simulink model "BMSOut"  (R2024b)
settings: configuration reference "VehicleFixed100ms" (kept outside this file)
undefined symbols (not defined in the file): PlntBattNumCellSer
settings Model: DataDictionary=VirtualVehicleTemplate.sldd  ModifiedByFormat=The MathWorks, Inc.  ExtModeTrigDuration=5  Creator=The MathWorks, Inc.  LastModifiedBy=The MathWorks, Inc.
settings ConfigSetRef: SourceName=VehicleFixed100ms

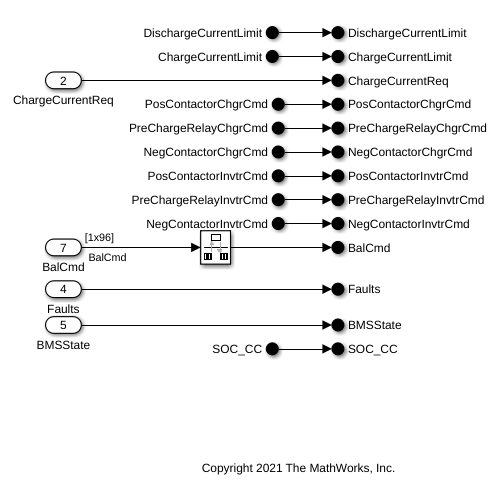
[thumbnail: Simulink's stored preview of the top-level diagram]
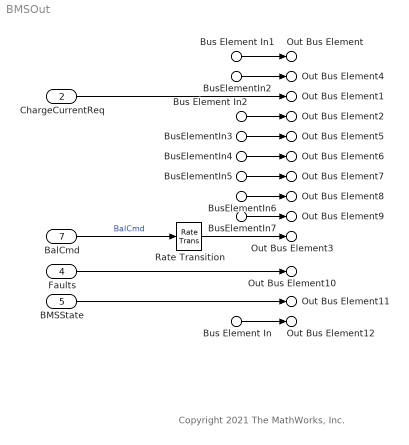
== system BMSOut ==
  note: Copyright 2021 The MathWorks, Inc.
  Bus Element In1 : Inport  PortName=CurrentLimits  Element=DischargeCurrentLimit
  BusElementIn2 : Inport  PortName=CurrentLimits  Element=ChargeCurrentLimit
  ChargeCurrentReq : Inport  Port=2  OutDataTypeStr=single  PortDimensions=1  SampleTime=[0.10000000000000001,0]
  Bus Element In2 : Inport  Port=3  PortName=Contactors_Cmd  Element=PosContactorChgrCmd
  BusElementIn3 : Inport  Port=3  PortName=Contactors_Cmd  Element=PreChargeRelayChgrCmd
  BusElementIn4 : Inport  Port=3  PortName=Contactors_Cmd  Element=NegContactorChgrCmd
  BusElementIn5 : Inport  Port=3  PortName=Contactors_Cmd  Element=PosContactorInvtrCmd
  BusElementIn6 : Inport  Port=3  PortName=Contactors_Cmd  Element=PreChargeRelayInvtrCmd
  BusElementIn7 : Inport  Port=3  PortName=Contactors_Cmd  Element=NegContactorInvtrCmd
  Faults : Inport  Port=4  OutDataTypeStr=boolean
  BMSState : Inport  Port=5  OutDataTypeStr=single  PortDimensions=1  SampleTime=[0.10000000000000001,0]
  Bus Element In : Inport  Port=6  PortName=SOC  Element=SOC_CC
  BalCmd : Inport  Port=7  OutDataTypeStr=boolean  PortDimensions=[1 PlntBattNumCellSer]  SampleTime=[5,0]
  Rate Transition : RateTransition  Integrity=off  Deterministic=off
  Out Bus Element : Outport  PortName=BMSCommands  Element=CurrentLimitsBus.DischargeCurrentLimit
  Out Bus Element4 : Outport  PortName=BMSCommands  Element=CurrentLimitsBus.ChargeCurrentLimit
  Out Bus Element1 : Outport  PortName=BMSCommands  Element=ChargeCurrentReq
  Out Bus Element2 : Outport  PortName=BMSCommands  Element=ContactorsCmdBus.PosContactorChgrCmd
  Out Bus Element5 : Outport  PortName=BMSCommands  Element=ContactorsCmdBus.PreChargeRelayChgrCmd
  Out Bus Element6 : Outport  PortName=BMSCommands  Element=ContactorsCmdBus.NegContactorChgrCmd
  Out Bus Element7 : Outport  PortName=BMSCommands  Element=ContactorsCmdBus.PosContactorInvtrCmd
  Out Bus Element8 : Outport  PortName=BMSCommands  Element=ContactorsCmdBus.PreChargeRelayInvtrCmd
  Out Bus Element9 : Outport  PortName=BMSCommands  Element=ContactorsCmdBus.NegContactorInvtrCmd
  Out Bus Element3 : Outport  PortName=BMSCommands  Element=BalCmd
  Out Bus Element10 : Outport  Port=2  PortName=BMSInfo  Element=Faults
  Out Bus Element11 : Outport  Port=2  PortName=BMSInfo  Element=BMSState
  Out Bus Element12 : Outport  Port=2  PortName=BMSInfo  Element=SOC.SOC_CC
  wires:
  BusElementIn4/1 -> Out Bus Element6/1
  Bus Element In2/1 -> Out Bus Element2/1
  BusElementIn2/1 -> Out Bus Element4/1
  BusElementIn3/1 -> Out Bus Element5/1
  BusElementIn6/1 -> Out Bus Element8/1
  ChargeCurrentReq/1 -> Out Bus Element1/1
  BusElementIn7/1 -> Out Bus Element9/1
  Rate Transition/1 -> Out Bus Element3/1
  BusElementIn5/1 -> Out Bus Element7/1
  BalCmd/1 -> Rate Transition/1  "BalCmd"
  BMSState/1 -> Out Bus Element11/1
  Faults/1 -> Out Bus Element10/1
  Bus Element In/1 -> Out Bus Element12/1
  Bus Element In1/1 -> Out Bus Element/1
